simulink library "qss_tb_library"  (Simulink 10.0)
settings: Solver=ode45  StartTime=0.0  StopTime=1220  RelTol=1e-3
undefined symbols (not defined in the file): automatic_gearbox, cc_done, delta_h_C_air, DiscIntNeverNeededParam, dw_GG_c, eta_EG_map, eta_EM_map, eta_ice, g, h, H_o_m, H_u, i_FC_in, i_FC_max, k1, k2, k3, k4, k_cs, M_air, manual_gearbox, P_aux, P_CE_cutoff, P_CE_idle, P_CE_recup, P_CVT_opt, Q_BT_min, Q_SC_IC, r, rho, rho_f, t_c, T_CE_cutoff, T_CE_max, T_EG_c, T_EG_max, T_EM_max, theta_CE, theta_EM, V_CE_map, V_FC_out, w_CE_idle, w_CE_max, w_CE_upper, w_CVT_opt, w_EG_row, w_EG_upper, w_EM_row, w_EM_upper, w_GG_c
(part 2 of 4)

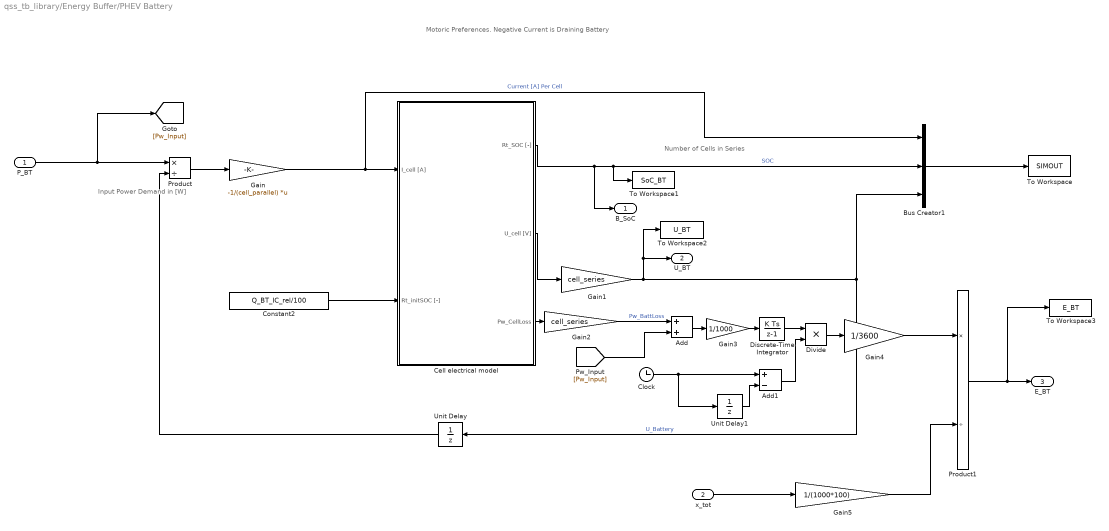
== system qss_tb_library/Energy Buffer/PHEV Battery ==
  note: Number of Cells in Series
  note: Motoric Preferences. Negative Current is Draining Battery
  note: Input Power Demand in [W]
  P_BT : Inport
  x_tot : Inport  Port=2
  Add : Sum
  Add1 : Sum  Inputs=+-
  Bus Creator1 : BusCreator  Inputs=3
  Cell electrical model : Subsystem
  Clock : Clock
  Constant2 : Constant  Value=Q_BT_IC_rel/100
  Discrete-Time Integrator : DiscreteIntegrator  ICPrevOutput=DiscIntNeverNeededParam  ICPrevScaledInput=DiscIntNeverNeededParam
  Divide : Product  Inputs=**
  Gain : Gain  Gain=-1/(cell_parallel)  Multiplication=Matrix(K*u)
  Gain1 : Gain  Gain=cell_series
  Gain2 : Gain  Gain=cell_series
  Gain3 : Gain  Gain=1/1000
  Gain4 : Gain  Gain=1/3600
  Gain5 : Gain  Gain=1/(1000*100)
  Product : Product  Inputs=*/  RndMeth=Zero
  Product1 : Product  Inputs=*/  SaturateOnIntegerOverflow=on  RndMeth=Zero  InputSameDT=on  OutDataTypeStr=Inherit: Same as first input
  To Workspace : ToWorkspace  VariableName=SIMOUT  SaveFormat=Structure With Time  SampleTime=-1
  To Workspace1 : ToWorkspace  VariableName=SoC_BT  SampleTime=-1
      settings: RequirementInfo={} %GIDa_c6642060_f8db_4366_a618_aa68098668f7
  To Workspace2 : ToWorkspace  VariableName=U_BT  SampleTime=-1
      settings: RequirementInfo={} %GIDa_32590376_96d5_473d_a7bc_23059799ede8
  To Workspace3 : ToWorkspace  VariableName=E_BT  SampleTime=-1
  Unit Delay : UnitDelay  InitialCondition=4.07*cell_series  HasFrameUpgradeWarning=on
  Unit Delay1 : UnitDelay  HasFrameUpgradeWarning=on
  B_SoC : Outport  InitialOutput=0
  U_BT : Outport  Port=2  InitialOutput=0
  E_BT : Outport  Port=3  InitialOutput=0
  wires:
  Add1/1 -> Divide/2
  Unit Delay1/1 -> Add1/2
  Clock/1 -> Add1/1, Unit Delay1/1
  Bus Creator1/1 -> To Workspace/1
  Discrete-Time Integrator/1 -> Divide/1
  x_tot/1 -> Gain5/1
  Gain5/1 -> Product1/2
  Gain4/1 -> Product1/1
  Divide/1 -> Gain4/1
  Gain3/1 -> Discrete-Time Integrator/1
  Add/1 -> Gain3/1
  [Pw_Input] -> Add/2
  Gain2/1 -> Add/1  "Pw_BattLoss"
  Cell electrical model/3(Pw_CellLoss) -> Gain2/1
  Product1/1 -> E_BT/1, To Workspace3/1
  P_BT/1 -> Product/1, [Pw_Input]
  Cell electrical model/1(Rt_SOC [-]) -> Bus Creator1/2, To Workspace1/1, B_SoC/1  "SOC"
  Unit Delay/1 -> Product/2
  Product/1 -> Gain/1
  Constant2/1 -> Cell electrical model/2(Rt_initSOC [-])
  Gain1/1 -> Unit Delay/1, Bus Creator1/3, U_BT/1, To Workspace2/1  "U_Battery"
  Cell electrical model/2(U_cell [V]) -> Gain1/1
  Gain/1 -> Cell electrical model/1(I_cell [A]), Bus Creator1/1  "Current [A] Per Cell"

== system qss_tb_library/Energy Buffer/Supercapacitor ==
  P_SC : Inport
  Fcn : Fcn  Expr=(-u[2]/C_SC+sqrt(u[2]^2/C_SC^2-4*R_SC*u[1]))/(2*R_SC)
  Gain : Gain  Gain=1/C_SC  SaturateOnIntegerOverflow=on  OutDataTypeStr=Inherit: Same as input  ParamDataTypeStr=Inherit: Same as input
  Gain1 : Gain  Gain=h  SaturateOnIntegerOverflow=on  OutDataTypeStr=Inherit: Same as input  ParamDataTypeStr=Inherit: Same as input
  Mux : Mux  Inputs=2
  SC charge : UnitDelay  InitialCondition=Q_SC_IC  SampleTime=h  HasFrameUpgradeWarning=on
  Sum3 : Sum  SaturateOnIntegerOverflow=on  InputSameDT=on  OutDataTypeStr=Inherit: Same as first input
  Supervision supercap : Subsystem
  To Workspace1 : ToWorkspace  VariableName=I_SC  SampleTime=1
  To Workspace2 : ToWorkspace  VariableName=U_SC  SampleTime=1
  To Workspace3 : ToWorkspace  VariableName=Q_SC  SampleTime=1
  To Workspace4 : ToWorkspace  VariableName=P_SC  SampleTime=1
  U_SC : Outport  InitialOutput=0
  wires:
  P_SC/1 -> Supervision supercap/2(P_SC), Mux/1, To Workspace4/1
  Gain/1 -> To Workspace2/1, U_SC/1
  Fcn/1 -> To Workspace1/1, Gain1/1
  SC charge/1 -> To Workspace3/1, Supervision supercap/1(Q_SC), Mux/2, Gain/1, Sum3/2
  Sum3/1 -> SC charge/1
  Mux/1 -> Fcn/1
  Gain1/1 -> Sum3/1

== system qss_tb_library/Energy Converter/CE Assignment ==
  w_gear : Inport
  dw_dt_gear : Inport  Port=2
  T_gear : Inport  Port=3
  Constant1 : Constant  Value=P_aux
  Detect fuel cutoff : Subsystem
  Detect idle : Subsystem
  Detect overload and overspeed : Subsystem
  "Engine consumption map V = f(w, T) [kg/s]" : Lookup2D  RowIndex=w_CE_row  ColumnIndex=T_CE_col  Table=V_CE_map
  Engine inertia : Gain  Gain=theta_CE  SaturateOnIntegerOverflow=on  OutDataTypeStr=Inherit: Same as input  ParamDataTypeStr=Inherit: Same as input
  Fuel lower heating value : Gain  Gain=H_u  SaturateOnIntegerOverflow=on  OutDataTypeStr=Inherit: Same as input  ParamDataTypeStr=Inherit: Same as input
  Lower limit (fuel cutoff) : Saturate  UpperLimit=inf  LowerLimit=T_CE_cutoff
  Lower limit (speed at idle) : Saturate  UpperLimit=inf  LowerLimit=w_CE_idle
  To Workspace3 : ToWorkspace  VariableName=T_CE  SampleTime=-1
  To Workspace4 : ToWorkspace  VariableName=w_CE  SampleTime=-1
  To Workspace5 : ToWorkspace  VariableName=P_CE  SampleTime=-1
  Total power : Sum  SaturateOnIntegerOverflow=on  InputSameDT=on  OutDataTypeStr=Inherit: Same as first input
  Total torque : Sum  SaturateOnIntegerOverflow=on  InputSameDT=on  OutDataTypeStr=Inherit: Same as first input
  P_CE : Outport  InitialOutput=0
  wires:
  Lower limit (fuel cutoff)/1 -> To Workspace3/1, Detect fuel cutoff/2(T_CE), Detect idle/3(T_CE), "Engine consumption map V = f(w, T) [kg/s]"/2, Detect overload and overspeed/2(T_CE)
  Constant1/1 -> Total power/2
  Total power/1 -> To Workspace5/1, P_CE/1
  Detect fuel cutoff/1(P_CE) -> Total power/1
  "Engine consumption map V = f(w, T) [kg/s]"/1 -> Fuel lower heating value/1
  Detect idle/1(P_CE) -> Detect fuel cutoff/1(P_CE_fuel)
  Fuel lower heating value/1 -> Detect idle/1(P_CE_fuel)
  w_gear/1 -> Lower limit (speed at idle)/1
  Lower limit (speed at idle)/1 -> To Workspace4/1, "Engine consumption map V = f(w, T) [kg/s]"/1, Detect idle/2(w_CE), Detect overload and overspeed/1(w_CE)
  Engine inertia/1 -> Total torque/2
  Total torque/1 -> Lower limit (fuel cutoff)/1
  dw_dt_gear/1 -> Engine inertia/1
  T_gear/1 -> Total torque/1

== system qss_tb_library/Energy Converter/Combustion Engine (Willans-approximation  with overload detection) ==
  w_gear : Inport
  dw_dt_gear : Inport  Port=2
  T_gear : Inport  Port=3
  Constant1 : Constant  Value=P_aux
  Detect fuel cutoff : Subsystem
  Detect idle : Subsystem
  Detect overload and overspeed : Subsystem
  Engine efficiency : Subsystem
  Engine inertia : Gain  Gain=theta_CE  SaturateOnIntegerOverflow=on  OutDataTypeStr=Inherit: Same as input  ParamDataTypeStr=Inherit: Same as input
  Lower limit (fuel cutoff) : Saturate  UpperLimit=inf  LowerLimit=T_CE_cutoff
  Lower limit (speed at idle) : Saturate  UpperLimit=inf  LowerLimit=w_CE_idle
  Product : Product  Inputs=**/  SaturateOnIntegerOverflow=on  RndMeth=Zero  InputSameDT=on  OutDataTypeStr=Inherit: Same as first input
  To Workspace1 : ToWorkspace  VariableName=eta_CE  SampleTime=-1
  To Workspace3 : ToWorkspace  VariableName=T_CE  SampleTime=-1
  To Workspace4 : ToWorkspace  VariableName=w_CE  SampleTime=-1
  To Workspace5 : ToWorkspace  VariableName=P_CE  SampleTime=-1
  Total power : Sum  SaturateOnIntegerOverflow=on  InputSameDT=on  OutDataTypeStr=Inherit: Same as first input
  Total torque : Sum  SaturateOnIntegerOverflow=on  InputSameDT=on  OutDataTypeStr=Inherit: Same as first input
  P_CE : Outport  InitialOutput=0
  wires:
  Constant1/1 -> Total power/2
  Total power/1 -> To Workspace5/1, P_CE/1
  Detect fuel cutoff/1(P_CE) -> Total power/1
  Detect idle/1(P_CE) -> Detect fuel cutoff/1(P_CE_fuel)
  Product/1 -> Detect idle/1(P_CE_fuel)
  w_gear/1 -> Lower limit (speed at idle)/1
  Lower limit (speed at idle)/1 -> Detect idle/2(w_CE), Engine efficiency/1(w_CE), Product/1, Detect overload and overspeed/1(w_CE), To Workspace4/1
  Lower limit (fuel cutoff)/1 -> To Workspace3/1, Engine efficiency/2(T_CE), Detect fuel cutoff/2(T_CE), Detect idle/3(T_CE), Product/2, Detect overload and overspeed/2(T_CE)
  Engine inertia/1 -> Total torque/2
  Total torque/1 -> Lower limit (fuel cutoff)/1
  dw_dt_gear/1 -> Engine inertia/1
  T_gear/1 -> Total torque/1
  Engine efficiency/1(eta_CE) -> To Workspace1/1, Product/3

== system qss_tb_library/Energy Converter/Combustion Engine (Willans-approximation) ==
  w_gear : Inport
  dw_dt_gear : Inport  Port=2
  T_gear : Inport  Port=3
  Constant1 : Constant  Value=P_aux
  Detect fuel cutoff : Subsystem
  Detect idle : Subsystem
  Engine efficiency : Subsystem
  Engine inertia : Gain  Gain=theta_CE  SaturateOnIntegerOverflow=on  OutDataTypeStr=Inherit: Same as input  ParamDataTypeStr=Inherit: Same as input
  Lower limit (fuel cutoff) : Saturate  UpperLimit=inf  LowerLimit=T_CE_cutoff
  Lower limit (speed at idle) : Saturate  UpperLimit=inf  LowerLimit=w_CE_idle
  Product : Product  Inputs=**/  SaturateOnIntegerOverflow=on  RndMeth=Zero  InputSameDT=on  OutDataTypeStr=Inherit: Same as first input
  To Workspace1 : ToWorkspace  VariableName=eta_CE  SampleTime=-1
  To Workspace3 : ToWorkspace  VariableName=T_CE  SampleTime=-1
  To Workspace4 : ToWorkspace  VariableName=w_CE  SampleTime=-1
  To Workspace5 : ToWorkspace  VariableName=P_CE  SampleTime=-1
  Total power : Sum  SaturateOnIntegerOverflow=on  InputSameDT=on  OutDataTypeStr=Inherit: Same as first input
  Total torque : Sum  SaturateOnIntegerOverflow=on  InputSameDT=on  OutDataTypeStr=Inherit: Same as first input
  P_CE : Outport  InitialOutput=0
  wires:
  Engine efficiency/1(eta_CE) -> Product/3, To Workspace1/1
  T_gear/1 -> Total torque/1
  dw_dt_gear/1 -> Engine inertia/1
  Total torque/1 -> Lower limit (fuel cutoff)/1
  Engine inertia/1 -> Total torque/2
  Lower limit (fuel cutoff)/1 -> Detect idle/3(T_CE), Detect fuel cutoff/2(T_CE), Engine efficiency/2(T_CE), Product/2, To Workspace3/1
  Lower limit (speed at idle)/1 -> To Workspace4/1, Engine efficiency/1(w_CE), Detect idle/2(w_CE), Product/1
  w_gear/1 -> Lower limit (speed at idle)/1
  Product/1 -> Detect idle/1(P_CE_fuel)
  Detect idle/1(P_CE) -> Detect fuel cutoff/1(P_CE_fuel)
  Detect fuel cutoff/1(P_CE) -> Total power/1
  Total power/1 -> P_CE/1, To Workspace5/1
  Constant1/1 -> Total power/2

== system qss_tb_library/Energy Converter/Combustion Engine (consumption map) ==
  w_gear : Inport
  dw_dt_gear : Inport  Port=2
  T_gear : Inport  Port=3
  Constant1 : Constant  Value=P_aux
  Detect fuel cutoff : Subsystem
  Detect idle : Subsystem
  Detect overload and overspeed : Subsystem
  "Engine consumption map V = f(w, T) [kg/s]" : Lookup2D  RowIndex=w_CE_row  ColumnIndex=T_CE_col  Table=V_CE_map
  Engine inertia : Gain  Gain=theta_CE  SaturateOnIntegerOverflow=on  OutDataTypeStr=Inherit: Same as input  ParamDataTypeStr=Inherit: Same as input
  Fuel lower heating value : Gain  Gain=H_u  SaturateOnIntegerOverflow=on  OutDataTypeStr=Inherit: Same as input  ParamDataTypeStr=Inherit: Same as input
  Lower limit (fuel cutoff) : Saturate  UpperLimit=inf  LowerLimit=T_CE_cutoff
  Lower limit (speed at idle) : Saturate  UpperLimit=inf  LowerLimit=w_CE_idle
  To Workspace3 : ToWorkspace  VariableName=T_CE  SampleTime=-1
  To Workspace4 : ToWorkspace  VariableName=w_CE  SampleTime=-1
  To Workspace5 : ToWorkspace  VariableName=P_CE  SampleTime=-1
  Total power : Sum  SaturateOnIntegerOverflow=on  InputSameDT=on  OutDataTypeStr=Inherit: Same as first input
  Total torque : Sum  SaturateOnIntegerOverflow=on  InputSameDT=on  OutDataTypeStr=Inherit: Same as first input
  P_CE : Outport  InitialOutput=0
  wires:
  T_gear/1 -> Total torque/1
  dw_dt_gear/1 -> Engine inertia/1
  Total torque/1 -> Lower limit (fuel cutoff)/1
  Engine inertia/1 -> Total torque/2
  Lower limit (speed at idle)/1 -> Detect overload and overspeed/1(w_CE), Detect idle/2(w_CE), "Engine consumption map V = f(w, T) [kg/s]"/1, To Workspace4/1
  w_gear/1 -> Lower limit (speed at idle)/1
  Fuel lower heating value/1 -> Detect idle/1(P_CE_fuel)
  Detect idle/1(P_CE) -> Detect fuel cutoff/1(P_CE_fuel)
  "Engine consumption map V = f(w, T) [kg/s]"/1 -> Fuel lower heating value/1
  Detect fuel cutoff/1(P_CE) -> Total power/1
  Total power/1 -> P_CE/1, To Workspace5/1
  Constant1/1 -> Total power/2
  Lower limit (fuel cutoff)/1 -> Detect overload and overspeed/2(T_CE), "Engine consumption map V = f(w, T) [kg/s]"/2, Detect idle/3(T_CE), Detect fuel cutoff/2(T_CE), To Workspace3/1

== system qss_tb_library/Energy Converter/Combustion Engine (ideal) ==
  w_gear : Inport
  dw_dt_gear : Inport  Port=2
  T_gear : Inport  Port=3
  Constant1 : Constant  Value=P_aux
  Efficiency : Gain  Gain=1/eta_ice  SaturateOnIntegerOverflow=on  OutDataTypeStr=Inherit: Same as input  ParamDataTypeStr=Inherit: Same as input
  Engine inertia : Gain  Gain=theta_CE  SaturateOnIntegerOverflow=on  OutDataTypeStr=Inherit: Same as input  ParamDataTypeStr=Inherit: Same as input
  Product : Product  RndMeth=Zero
  To Workspace3 : ToWorkspace  VariableName=T_CE  SampleTime=-1
  To Workspace4 : ToWorkspace  VariableName=w_CE  SampleTime=-1
  To Workspace5 : ToWorkspace  VariableName=P_CE  SampleTime=-1
  Total power : Sum  Inputs=+++  SaturateOnIntegerOverflow=on  InputSameDT=on  OutDataTypeStr=Inherit: Same as first input
  Total torque : Sum  SaturateOnIntegerOverflow=on  InputSameDT=on  OutDataTypeStr=Inherit: Same as first input
  "idle -> inf" : Saturate  UpperLimit=inf  LowerLimit=P_CE_idle
  recuperation : Saturate  UpperLimit=0  LowerLimit=P_CE_recup
  P_CE : Outport  InitialOutput=0
  wires:
  recuperation/1 -> Total power/3
  "idle -> inf"/1 -> Efficiency/1
  Constant1/1 -> Total power/2
  Total power/1 -> To Workspace5/1, P_CE/1
  Efficiency/1 -> Total power/1
  Product/1 -> recuperation/1, "idle -> inf"/1
  w_gear/1 -> To Workspace4/1, Product/1
  Engine inertia/1 -> Total torque/2
  Total torque/1 -> To Workspace3/1, Product/2
  dw_dt_gear/1 -> Engine inertia/1
  T_gear/1 -> Total torque/1

== system qss_tb_library/Energy Converter/EG Assignment ==
  w_gear : Inport
  T_gear : Inport  Port=2
  Detect overload and overspeed : Subsystem
  "Efficiency eta = f(w, T)" : Lookup2D  RowIndex=w_EG_row  ColumnIndex=T_EG_col  Table=eta_EG_map
  Product : Product  Inputs=3  SaturateOnIntegerOverflow=on  RndMeth=Zero  InputSameDT=on  OutDataTypeStr=Inherit: Same as first input
  To Workspace1 : ToWorkspace  VariableName=w_EG  SampleTime=-1
  To Workspace2 : ToWorkspace  VariableName=T_EG  SampleTime=-1
  To Workspace5 : ToWorkspace  VariableName=P_EG  SampleTime=-1
  P_EG : Outport  InitialOutput=0
  wires:
  T_gear/1 -> Product/2, "Efficiency eta = f(w, T)"/2, Detect overload and overspeed/2(T_EG), To Workspace2/1
  "Efficiency eta = f(w, T)"/1 -> Product/1
  Product/1 -> P_EG/1, To Workspace5/1
  w_gear/1 -> Product/3, "Efficiency eta = f(w, T)"/1, Detect overload and overspeed/1(w_EG), To Workspace1/1

== system qss_tb_library/Energy Converter/EM Assignment ==
  w_gear : Inport
  dw_dt_gear : Inport  Port=2
  T_gear : Inport  Port=3
  Constant1 : Constant  Value=P_aux
  Detect overload and overspeed : Subsystem
  "Efficiency eta = f(w, T)" : Lookup2D  RowIndex=w_EM_row  ColumnIndex=T_EM_col  Table=eta_EM_map
  Gain1 : Gain  Gain=theta_EM  SaturateOnIntegerOverflow=on  OutDataTypeStr=Inherit: Same as input  ParamDataTypeStr=Inherit: Same as input
  Product : Product  Inputs=3  SaturateOnIntegerOverflow=on  RndMeth=Zero  InputSameDT=on  OutDataTypeStr=Inherit: Same as first input
  To Workspace1 : ToWorkspace  VariableName=w_EM  SampleTime=-1
  To Workspace2 : ToWorkspace  VariableName=T_EM  SampleTime=-1
  To Workspace5 : ToWorkspace  VariableName=P_EM  SampleTime=-1
  Total power : Sum  SaturateOnIntegerOverflow=on  InputSameDT=on  OutDataTypeStr=Inherit: Same as first input
  Total torque : Sum  SaturateOnIntegerOverflow=on  InputSameDT=on  OutDataTypeStr=Inherit: Same as first input
  P_EM : Outport  InitialOutput=0
  wires:
  w_gear/1 -> Detect overload and overspeed/1(w_EM), "Efficiency eta = f(w, T)"/1, Product/3, To Workspace1/1
  "Efficiency eta = f(w, T)"/1 -> Product/1
  dw_dt_gear/1 -> Gain1/1
  T_gear/1 -> Total torque/2
  Gain1/1 -> Total torque/1
  Total torque/1 -> Detect overload and overspeed/2(T_EM), "Efficiency eta = f(w, T)"/2, Product/2, To Workspace2/1
  Constant1/1 -> Total power/2
  Product/1 -> Total power/1
  Total power/1 -> P_EM/1, To Workspace5/1

== system qss_tb_library/Energy Converter/Electric Generator ==
  w_gear : Inport
  T_gear : Inport  Port=2
  Detect overload and overspeed : Subsystem
  "Efficiency eta = f(w, T)" : Lookup2D  RowIndex=w_EG_row  ColumnIndex=T_EG_col  Table=eta_EG_map
  Product : Product  Inputs=3  SaturateOnIntegerOverflow=on  RndMeth=Zero  InputSameDT=on  OutDataTypeStr=Inherit: Same as first input
  To Workspace1 : ToWorkspace  VariableName=w_EG  SampleTime=-1
  To Workspace2 : ToWorkspace  VariableName=T_EG  SampleTime=-1
  To Workspace5 : ToWorkspace  VariableName=P_EG  SampleTime=-1
  P_EG : Outport  InitialOutput=0
  wires:
  T_gear/1 -> Product/2, "Efficiency eta = f(w, T)"/2, Detect overload and overspeed/2(T_EG), To Workspace2/1
  "Efficiency eta = f(w, T)"/1 -> Product/1
  Product/1 -> P_EG/1, To Workspace5/1
  w_gear/1 -> Product/3, "Efficiency eta = f(w, T)"/1, Detect overload and overspeed/1(w_EG), To Workspace1/1

== system qss_tb_library/Energy Converter/Electric Motor ==
  w_gear : Inport
  dw_dt_gear : Inport  Port=2
  T_gear : Inport  Port=3
  Constant1 : Constant  Value=P_aux
  Detect overload and overspeed : Subsystem
  "Efficiency eta = f(w, T)" : Lookup2D  RowIndex=w_EM_row  ColumnIndex=T_EM_col  Table=eta_EM_map
  Gain1 : Gain  Gain=theta_EM  SaturateOnIntegerOverflow=on  OutDataTypeStr=Inherit: Same as input  ParamDataTypeStr=Inherit: Same as input
  Product : Product  Inputs=3  SaturateOnIntegerOverflow=on  RndMeth=Zero  InputSameDT=on  OutDataTypeStr=Inherit: Same as first input
  To Workspace1 : ToWorkspace  VariableName=w_EM  SampleTime=-1
  To Workspace2 : ToWorkspace  VariableName=T_EM  SampleTime=-1
  To Workspace5 : ToWorkspace  VariableName=P_EM  SampleTime=-1
  Total power : Sum  SaturateOnIntegerOverflow=on  InputSameDT=on  OutDataTypeStr=Inherit: Same as first input
  Total torque : Sum  SaturateOnIntegerOverflow=on  InputSameDT=on  OutDataTypeStr=Inherit: Same as first input
  P_EM : Outport  InitialOutput=0
  wires:
  w_gear/1 -> Detect overload and overspeed/1(w_EM), "Efficiency eta = f(w, T)"/1, Product/3, To Workspace1/1
  "Efficiency eta = f(w, T)"/1 -> Product/1
  dw_dt_gear/1 -> Gain1/1
  T_gear/1 -> Total torque/2
  Gain1/1 -> Total torque/1
  Total torque/1 -> Detect overload and overspeed/2(T_EM), "Efficiency eta = f(w, T)"/2, Product/2, To Workspace2/1
  Constant1/1 -> Total power/2
  Product/1 -> Total power/1
  Total power/1 -> P_EM/1, To Workspace5/1

== system qss_tb_library/Energy Converter/Fuel Cell ==
  note: E-Motor is disengaged, as soon as required power
      |  is <= P_fc_idle (->idle speed energy consumption)
  P_in : Inport
  Compressor with E-motor : Subsystem
  Constant3 : Constant  Value=P_FC_idle
  Constant4 : Constant  Value=V_th
  Fuel cell model : Lookup  InputValues=i_FC_in  Table=V_FC_out  SaturateOnIntegerOverflow=on
  Heat losses : ToWorkspace  VariableName=P_loss  SampleTime=1
  Product2 : Product  SaturateOnIntegerOverflow=on  RndMeth=Zero  InputSameDT=on  OutDataTypeStr=Inherit: Same as first input
  Product3 : Product  Inputs=/*  SaturateOnIntegerOverflow=on  RndMeth=Zero  InputSameDT=on  OutDataTypeStr=Inherit: Same as first input
  Stack current : Product  Inputs=*/  SaturateOnIntegerOverflow=on  RndMeth=Zero  InputSameDT=on  OutDataTypeStr=Inherit: Same as first input
  Stack voltage : UnitDelay  InitialCondition=10  SampleTime=h  HasFrameUpgradeWarning=on
  Sum : Sum  SaturateOnIntegerOverflow=on  InputSameDT=on  OutDataTypeStr=Inherit: Same as first input
  Sum1 : Sum  Inputs=+-  SaturateOnIntegerOverflow=on  InputSameDT=on  OutDataTypeStr=Inherit: Same as first input
  Supervision of current density : Subsystem
  Switch1 : Switch  Threshold=P_FC_idle  SaturateOnIntegerOverflow=on  InputSameDT=on
  Theoretical cell voltage : Gain  Gain=1/V_th  SaturateOnIntegerOverflow=on  OutDataTypeStr=Inherit: Same as input  ParamDataTypeStr=Inherit: Same as input
  To Workspace2 : ToWorkspace  VariableName=V_FC  SampleTime=1
  To Workspace4 : ToWorkspace  VariableName=I_FC  SampleTime=1
  To Workspace5 : ToWorkspace  VariableName=i_FC  SampleTime=1
  To Workspace7 : ToWorkspace  VariableName=P_FC  SampleTime=1
  "[A/m^2]" : Gain  Gain=1/A_FC  SaturateOnIntegerOverflow=on  OutDataTypeStr=Inherit: Same as input  ParamDataTypeStr=Inherit: Same as input
  stack number : Gain  Gain=N_FC  SaturateOnIntegerOverflow=on  OutDataTypeStr=Inherit: Same as input  ParamDataTypeStr=Inherit: Same as input
  stack number1 : Gain  Gain=N_FC  SaturateOnIntegerOverflow=on  OutDataTypeStr=Inherit: Same as input  ParamDataTypeStr=Inherit: Same as input
  P_FC : Outport  InitialOutput=0
  wires:
  Compressor with E-motor/1(P_EM_C) -> Sum/2
  Switch1/1 -> Stack current/1, Product3/2
  Constant3/1 -> Switch1/3
  Sum/1 -> Switch1/2, Switch1/1
  P_in/1 -> Sum/1
  Constant4/1 -> Sum1/1
  stack number/1 -> Stack voltage/1
  Sum1/1 -> stack number1/1
  stack number1/1 -> Product2/2
  "[A/m^2]"/1 -> Fuel cell model/1, To Workspace5/1, Supervision of current density/1("   i_FC")
  Theoretical cell voltage/1 -> Product3/1
  Fuel cell model/1 -> stack number/1, Sum1/2, Theoretical cell voltage/1
  Stack current/1 -> "[A/m^2]"/1, Product2/1, To Workspace4/1
  Stack voltage/1 -> Stack current/2, To Workspace2/1
  Product3/1 -> P_FC/1, To Workspace7/1, Compressor with E-motor/1(P_FC)
  Product2/1 -> Heat losses/1

== system qss_tb_library/Energy Source/Tank ==
  P_fuel : Inport
  x_tot : Inport  Port=2
  Factor for cold start : Gain  Gain=k_cs  SaturateOnIntegerOverflow=on  OutDataTypeStr=Inherit: Same as input  ParamDataTypeStr=Inherit: Same as input
  Fu2131el density : Gain  Gain=1/rho_f  SaturateOnIntegerOverflow=on  OutDataTypeStr=Inherit: Same as input  ParamDataTypeStr=Inherit: Same as input
  Gain3 : Gain  Gain=1e5  SaturateOnIntegerOverflow=on  OutDataTypeStr=Inherit: Same as input  ParamDataTypeStr=Inherit: Same as input
  Integration : Subsystem
  Product : Product  Inputs=*/  SaturateOnIntegerOverflow=on  RndMeth=Zero  InputSameDT=on  OutDataTypeStr=Inherit: Same as first input
  To Workspace7 : ToWorkspace  VariableName=V_liter  SampleTime=-1
  liter/100 km : Outport  InitialOutput=0
  wires:
  P_fuel/1 -> Integration/1(P_fuel)
  x_tot/1 -> Product/2
  Integration/1(m_fuel) -> Fu2131el density/1
  Gain3/1 -> liter/100 km/1, To Workspace7/1
  Fu2131el density/1 -> Product/1
  Product/1 -> Factor for cold start/1
  Factor for cold start/1 -> Gain3/1

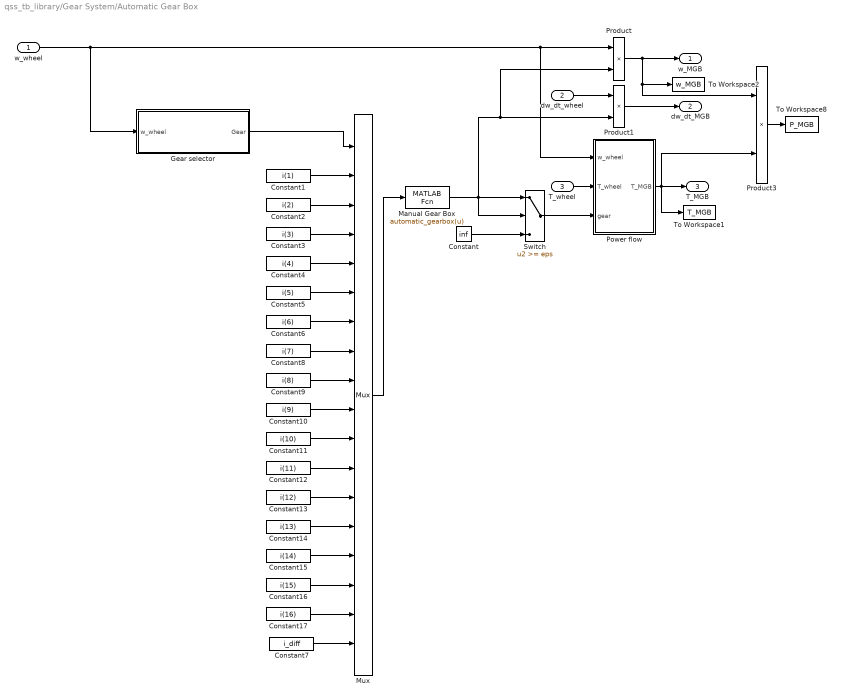
== system qss_tb_library/Gear System/Automatic Gear Box ==
  w_wheel : Inport
  dw_dt_wheel : Inport  Port=2
  T_wheel : Inport  Port=3
  Constant : Constant  Value=inf
  Constant1 : Constant  Value=i(1)
  Constant10 : Constant  Value=i(9)
  Constant11 : Constant  Value=i(10)
  Constant12 : Constant  Value=i(11)
  Constant13 : Constant  Value=i(12)
  Constant14 : Constant  Value=i(13)
  Constant15 : Constant  Value=i(14)
  Constant16 : Constant  Value=i(15)
  Constant17 : Constant  Value=i(16)
  Constant2 : Constant  Value=i(2)
  Constant3 : Constant  Value=i(3)
  Constant4 : Constant  Value=i(4)
  Constant5 : Constant  Value=i(5)
  Constant6 : Constant  Value=i(6)
  Constant7 : Constant  Value=i_diff
  Constant8 : Constant  Value=i(7)
  Constant9 : Constant  Value=i(8)
  Gear selector : Subsystem
  Manual Gear Box : MATLABFcn  MATLABFcn=automatic_gearbox(u)  OutputDimensions=1
  Mux : Mux  Inputs=18
  Power flow : Subsystem
  Product : Product  SaturateOnIntegerOverflow=on  RndMeth=Zero  InputSameDT=on  OutDataTypeStr=Inherit: Same as first input
  Product1 : Product  SaturateOnIntegerOverflow=on  RndMeth=Zero  InputSameDT=on  OutDataTypeStr=Inherit: Same as first input
  Product3 : Product  SaturateOnIntegerOverflow=on  RndMeth=Zero  InputSameDT=on  OutDataTypeStr=Inherit: Same as first input
  Switch : Switch  Threshold=eps  SaturateOnIntegerOverflow=on  InputSameDT=on
  To Workspace1 : ToWorkspace  VariableName=T_MGB  SampleTime=-1
  To Workspace2 : ToWorkspace  VariableName=w_MGB  SampleTime=-1
  To Workspace8 : ToWorkspace  VariableName=P_MGB  SampleTime=-1
  w_MGB : Outport  InitialOutput=0
  dw_dt_MGB : Outport  Port=2  InitialOutput=0
  T_MGB : Outport  Port=3  InitialOutput=0
  wires:
  Mux/1 -> Manual Gear Box/1
  Gear selector/1(Gear) -> Mux/1
  Constant6/1 -> Mux/7
  Constant5/1 -> Mux/6
  Constant4/1 -> Mux/5
  Constant3/1 -> Mux/4
  Constant2/1 -> Mux/3
  Constant1/1 -> Mux/2
  T_wheel/1 -> Power flow/2(T_wheel)
  Switch/1 -> Power flow/3(gear)
  Product3/1 -> To Workspace8/1
  Manual Gear Box/1 -> Switch/1, Switch/2, Product1/2, Product/2
  dw_dt_wheel/1 -> Product1/1
  Product1/1 -> dw_dt_MGB/1
  w_wheel/1 -> Power flow/1(w_wheel), Product/1, Gear selector/1(w_wheel)
  Constant/1 -> Switch/3
  Product/1 -> To Workspace2/1, Product3/1, w_MGB/1
  Power flow/1(T_MGB) -> To Workspace1/1, Product3/2, T_MGB/1
  Constant7/1 -> Mux/18
  Constant8/1 -> Mux/8
  Constant9/1 -> Mux/9
  Constant10/1 -> Mux/10
  Constant11/1 -> Mux/11
  Constant12/1 -> Mux/12
  Constant13/1 -> Mux/13
  Constant14/1 -> Mux/14
  Constant15/1 -> Mux/15
  Constant16/1 -> Mux/16
  Constant17/1 -> Mux/17

== system qss_tb_library/Gear System/Continuously Variable Transmission ==
  w_wheel : Inport
  dw_dt_wheel : Inport  Port=2
  T_wheel : Inport  Port=3
  j_CVT : Inport  Port=4
  dj_CVT : Inport  Port=5
  Power flow : Subsystem
  Product{,1..3} (4 alike) : Product  SaturateOnIntegerOverflow=on  RndMeth=Zero  InputSameDT=on  OutDataTypeStr=Inherit: Same as first input
  Sum : Sum  SaturateOnIntegerOverflow=on  InputSameDT=on  OutDataTypeStr=Inherit: Same as first input
  To Workspace1 : ToWorkspace  VariableName=w_CVT  SampleTime=-1
  To Workspace8 : ToWorkspace  VariableName=P_CVT  SampleTime=-1
  To Workspace9 : ToWorkspace  VariableName=T_CVT  SampleTime=-1
  w_CVT : Outport  InitialOutput=0
  dw_dt_CVT : Outport  Port=2  InitialOutput=0
  T_CVT : Outport  Port=3  InitialOutput=0
  wires:
  w_wheel/1 -> Power flow/1(w_wheel), Product2/1, Product/1
  Power flow/1(T_CVT) -> To Workspace9/1, T_CVT/1, Product3/2
  Product/1 -> Product3/1, w_CVT/1, To Workspace1/1
  Sum/1 -> dw_dt_CVT/1
  dw_dt_wheel/1 -> Product1/1
  dj_CVT/1 -> Product2/2
  j_CVT/1 -> Product1/2, Product/2, Power flow/3(j_CVT)
  Product1/1 -> Sum/2
  Product2/1 -> Sum/1
  T_wheel/1 -> Power flow/2(T_wheel)
  Product3/1 -> To Workspace8/1

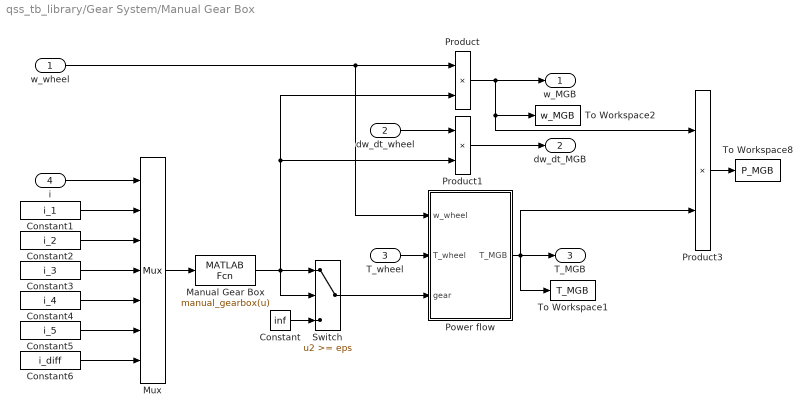
== system qss_tb_library/Gear System/Manual Gear Box ==
  w_wheel : Inport
  dw_dt_wheel : Inport  Port=2
  T_wheel : Inport  Port=3
  i : Inport  Port=4
  Constant : Constant  Value=inf
  Constant1 : Constant  Value=i_1
  Constant2 : Constant  Value=i_2
  Constant3 : Constant  Value=i_3
  Constant4 : Constant  Value=i_4
  Constant5 : Constant  Value=i_5
  Constant6 : Constant  Value=i_diff
  Manual Gear Box : MATLABFcn  MATLABFcn=manual_gearbox(u)  OutputDimensions=1
  Mux : Mux  Inputs=7
  Power flow : Subsystem
  Product : Product  SaturateOnIntegerOverflow=on  RndMeth=Zero  InputSameDT=on  OutDataTypeStr=Inherit: Same as first input
  Product1 : Product  SaturateOnIntegerOverflow=on  RndMeth=Zero  InputSameDT=on  OutDataTypeStr=Inherit: Same as first input
  Product3 : Product  SaturateOnIntegerOverflow=on  RndMeth=Zero  InputSameDT=on  OutDataTypeStr=Inherit: Same as first input
  Switch : Switch  Threshold=eps  SaturateOnIntegerOverflow=on  InputSameDT=on
  To Workspace1 : ToWorkspace  VariableName=T_MGB  SampleTime=-1
  To Workspace2 : ToWorkspace  VariableName=w_MGB  SampleTime=-1
  To Workspace8 : ToWorkspace  VariableName=P_MGB  SampleTime=-1
  w_MGB : Outport  InitialOutput=0
  dw_dt_MGB : Outport  Port=2  InitialOutput=0
  T_MGB : Outport  Port=3  InitialOutput=0
  wires:
  Power flow/1(T_MGB) -> T_MGB/1, Product3/2, To Workspace1/1
  Product/1 -> w_MGB/1, Product3/1, To Workspace2/1
  Constant/1 -> Switch/3
  w_wheel/1 -> Product/1, Power flow/1(w_wheel)
  Product1/1 -> dw_dt_MGB/1
  dw_dt_wheel/1 -> Product1/1
  Manual Gear Box/1 -> Product/2, Product1/2, Switch/2, Switch/1
  Product3/1 -> To Workspace8/1
  Switch/1 -> Power flow/3(gear)
  T_wheel/1 -> Power flow/2(T_wheel)
  Constant1/1 -> Mux/2
  Constant2/1 -> Mux/3
  Constant3/1 -> Mux/4
  Constant4/1 -> Mux/5
  Constant5/1 -> Mux/6
  Constant6/1 -> Mux/7
  i/1 -> Mux/1
  Mux/1 -> Manual Gear Box/1

== system qss_tb_library/Gear System/Simple Transmission ==
  w_wheel : Inport
  dw_dt_wheel : Inport  Port=2
  t_wheel : Inport  Port=3
  Constant : Constant  Value=gear_ratio
  Power flow : Subsystem
  Product : Product  SaturateOnIntegerOverflow=on  RndMeth=Zero  InputSameDT=on  OutDataTypeStr=Inherit: Same as first input
  Product1 : Product  SaturateOnIntegerOverflow=on  RndMeth=Zero  InputSameDT=on  OutDataTypeStr=Inherit: Same as first input
  Product3 : Product  SaturateOnIntegerOverflow=on  RndMeth=Zero  InputSameDT=on  OutDataTypeStr=Inherit: Same as first input
  To Workspace1 : ToWorkspace  VariableName=w_trans  SampleTime=-1
  To Workspace2 : ToWorkspace  VariableName=T_trans  SampleTime=-1
  To Workspace3 : ToWorkspace  VariableName=P_trans  SampleTime=-1
  w_trans : Outport  InitialOutput=0
  dw_dt_trans : Outport  Port=2  InitialOutput=0
  T_trans : Outport  Port=3  InitialOutput=0
  wires:
  Product3/1 -> To Workspace3/1
  Constant/1 -> Product/2, Product1/2, Power flow/3(gear_ratio)
  dw_dt_wheel/1 -> Product1/1
  Product/1 -> Product3/1, To Workspace1/1, w_trans/1
  Product1/1 -> dw_dt_trans/1
  Power flow/1(T_trans) -> Product3/2, To Workspace2/1, T_trans/1
  w_wheel/1 -> Power flow/1(w_wheel), Product/1
  t_wheel/1 -> Power flow/2(T_wheel)

== system qss_tb_library/Gear System/Simple Transmission2 ==
  w_wheel : Inport
  dw_dt_wheel : Inport  Port=2
  T_wheel : Inport  Port=3
  Product3 : Product  SaturateOnIntegerOverflow=on  RndMeth=Zero  InputSameDT=on  OutDataTypeStr=Inherit: Same as first input
  To Workspace1 : ToWorkspace  VariableName=w_trans  SampleTime=-1
  To Workspace2 : ToWorkspace  VariableName=T_trans  SampleTime=-1
  To Workspace3 : ToWorkspace  VariableName=P_trans  SampleTime=-1
  w_trans : Outport  InitialOutput=0
  dw_dt_trans : Outport  Port=2  InitialOutput=0
  T_trans : Outport  Port=3  InitialOutput=0
  wires:
  dw_dt_wheel/1 -> dw_dt_trans/1
  T_wheel/1 -> To Workspace2/1, T_trans/1, Product3/2
  w_wheel/1 -> w_trans/1, Product3/1, To Workspace1/1
  Product3/1 -> To Workspace3/1

== system qss_tb_library/Vehicle/Simple wheel model ==
  v_veh : Inport
  a_veh : Inport  Port=2
  F_Trac : Inport  Port=3
  Gain1 : Gain  Gain=1/(0.5*d_wheel)  SaturateOnIntegerOverflow=on  OutDataTypeStr=Inherit: Same as input  ParamDataTypeStr=Inherit: Same as input
  Gain2 : Gain  Gain=1/(0.5*d_wheel)  SaturateOnIntegerOverflow=on  OutDataTypeStr=Inherit: Same as input  ParamDataTypeStr=Inherit: Same as input
  Gain3 : Gain  Gain=0.5*d_wheel  SaturateOnIntegerOverflow=on  OutDataTypeStr=Inherit: Same as input  ParamDataTypeStr=Inherit: Same as input
  To Workspace1 : ToWorkspace  VariableName=w_wheel  SampleTime=-1
  To Workspace2 : ToWorkspace  VariableName=T_wheel  SampleTime=-1
  To Workspace3 : ToWorkspace  VariableName=dw_dt_wheel  SampleTime=-1
  w_wheel : Outport  InitialOutput=0
  dw_dt_wheel : Outport  Port=2  InitialOutput=0
  T_wheel : Outport  Port=3  InitialOutput=0
  wires:
  Gain2/1 -> dw_dt_wheel/1, To Workspace3/1
  Gain1/1 -> w_wheel/1, To Workspace1/1
  Gain3/1 -> To Workspace2/1, T_wheel/1
  a_veh/1 -> Gain2/1
  F_Trac/1 -> Gain3/1
  v_veh/1 -> Gain1/1

== system qss_tb_library/Vehicle/Vehicle ==
  v : Inport
  a : Inport  Port=2
  alfa : Inport  Port=3
  Acceleration Force : Subsystem
  Aerodynamic resistance : Subsystem
  Average speed : Subsystem
  Gain1 : Gain  Gain=1+k_inertia/100  SaturateOnIntegerOverflow=on  OutDataTypeStr=Inherit: Same as input  ParamDataTypeStr=Inherit: Same as input
  Required Traction force : Sum  Inputs=++++  SaturateOnIntegerOverflow=on  InputSameDT=on  OutDataTypeStr=Inherit: Same as first input
  Rolling resistance : Subsystem
  To Workspace1 : ToWorkspace  VariableName=v_veh  SampleTime=-1
  To Workspace2 : ToWorkspace  VariableName=F_grade  SampleTime=-1
  To Workspace3 : ToWorkspace  VariableName=a_veh  SampleTime=-1
  To Workspace5 : ToWorkspace  VariableName=F_roll  SampleTime=-1
  To Workspace6 : ToWorkspace  VariableName=F_Trac  SampleTime=-1
  To Workspace8 : ToWorkspace  VariableName=F_net  SampleTime=-1
  To Workspace9 : ToWorkspace  VariableName=F_aero  SampleTime=-1
  gradient force : Subsystem
  v_veh : Outport  InitialOutput=0
  a_veh : Outport  Port=2  InitialOutput=0
  F_Trac : Outport  Port=3  InitialOutput=0
  wires:
  Gain1/1 -> Required Traction force/3, To Workspace8/1
  gradient force/1(F_grade) -> To Workspace2/1, Required Traction force/4
  alfa/1 -> gradient force/1(alfa), Rolling resistance/2(alfa)
  Required Traction force/1 -> F_Trac/1, To Workspace6/1
  Acceleration Force/1(F_Net) -> Gain1/1
  Aerodynamic resistance/1(F_aero) -> To Workspace9/1, Required Traction force/2
  Rolling resistance/1(F_roll) -> To Workspace5/1, Required Traction force/1
  a/1 -> Acceleration Force/1(a_veh), To Workspace3/1, a_veh/1
  v/1 -> Average speed/1(v)
  Average speed/1(v_a) -> Aerodynamic resistance/1(v), Rolling resistance/1(v), v_veh/1, To Workspace1/1

== system qss_tb_library/Controller/Battery Controller/Geno-Group On ==
  cc_on : Inport
  Clock : Subsystem  mask(Digital clock){Parameter2=2}
      mask prompts: Parameter2 "Period:"
      mask help:
      | Digital clock.
      | Output is set to 1 for the first half of the period.
      mask init:
      | duration = @1/2;
      mask Help: Digital clock for logic systems.
      mask Display: plot(0,0,100,100,[90,75,75,60,60,35,35,20,20,10],[20,20,80,80,19,20,80,80,20,20])
  Constant : Constant  Value=cc_done
  Counter : UnitDelay  SampleTime=h  HasFrameUpgradeWarning=on
  Data Type Conversion1 : DataTypeConversion  OutDataTypeStr=boolean
  Data Type Conversion2 : DataTypeConversion  OutDataTypeStr=double
  Data Type Conversion3 : DataTypeConversion  OutDataTypeStr=double
  Logical operator3 : Logic
  Mux : Mux  Inputs=3
  Product : Product  SaturateOnIntegerOverflow=on  RndMeth=Zero  InputSameDT=on  OutDataTypeStr=Inherit: Same as first input
  Relational Operator : RelationalOperator  OutDataTypeStr=boolean  RndMeth=Nearest  InputSameDT=on
  Sum3 : Sum  Inputs=++-  SaturateOnIntegerOverflow=on  InputSameDT=on  OutDataTypeStr=Inherit: Same as first input
  T_EG start-up : Lookup  InputValues=t_c  Table=T_EG_c  SaturateOnIntegerOverflow=on
  dw start-up : Lookup  InputValues=t_c  Table=dw_GG_c  SaturateOnIntegerOverflow=on
  w start-up : Lookup  InputValues=t_c  Table=w_GG_c  SaturateOnIntegerOverflow=on
  OutOn : Outport  InitialOutput=0
  done : Outport  Port=2  InitialOutput=0
  wires:
  Data Type Conversion3/1 -> Product/1
  Data Type Conversion2/1 -> Sum3/2
  Data Type Conversion1/1 -> Logical operator3/2
  Mux/1 -> OutOn/1
  T_EG start-up/1 -> Mux/3
  dw start-up/1 -> Mux/2
  w start-up/1 -> Mux/1
  Logical operator3/1 -> Data Type Conversion2/1
  Counter/1 -> Sum3/1, dw start-up/1, T_EG start-up/1, Product/2, Relational Operator/1, w start-up/1
  Sum3/1 -> Counter/1
  Clock/1(out_1) -> Data Type Conversion1/1
  cc_on/1 -> Logical operator3/1
  Product/1 -> Sum3/3
  Constant/1 -> Relational Operator/2
  Relational Operator/1 -> Data Type Conversion3/1, done/1

== system qss_tb_library/Controller/Battery Controller/S-R Flip-Flop ==
  S : Inport
  R : Inport  Port=2
  Demux : Demux  Outputs=2
  Logic : CombinatorialLogic  TruthTable=[0 1;0 1;1 0;0 1;1 0;0 1;1 0;1 0]
  Memory : Memory  InheritSampleTime=on
  Mux : Mux  Inputs=3
  Q : Outport  InitialOutput=0
  !Q : Outport  Port=2  InitialOutput=1
  wires:
  R/1 -> Mux/3
  S/1 -> Mux/2
  Memory/1 -> Mux/1
  Demux/1 -> Memory/1, Q/1
  Demux/2 -> !Q/1
  Logic/1 -> Demux/1
  Mux/1 -> Logic/1

== system qss_tb_library/Driving Cycle/Driving Cycle/Differentiation ==
  V_z : Inport
  Sum1 : Sum  Inputs=+-  SaturateOnIntegerOverflow=on  InputSameDT=on  OutDataTypeStr=Inherit: Same as first input
  Unit Delay1 : UnitDelay  SampleTime=h  HasFrameUpgradeWarning=on
  D_z : Outport  InitialOutput=0
  wires:
  Sum1/1 -> D_z/1
  V_z/1 -> Unit Delay1/1, Sum1/1
  Unit Delay1/1 -> Sum1/2

== system qss_tb_library/Driving Cycle/Driving Cycle/Integration ==
  V_z : Inport
  Gain4 : Gain  Gain=0.5*h  SaturateOnIntegerOverflow=on  OutDataTypeStr=Inherit: Same as input  ParamDataTypeStr=Inherit: Same as input
  Plant : UnitDelay  InitialCondition=1  SampleTime=h  HasFrameUpgradeWarning=on
  Sum2 : Sum  SaturateOnIntegerOverflow=on  InputSameDT=on  OutDataTypeStr=Inherit: Same as first input
  Sum4 : Sum  SaturateOnIntegerOverflow=on  InputSameDT=on  OutDataTypeStr=Inherit: Same as first input
  Unit Delay2 : UnitDelay  SampleTime=h  HasFrameUpgradeWarning=on
  x_tot : Outport  InitialOutput=0
  wires:
  Plant/1 -> x_tot/1, Sum4/1
  Sum4/1 -> Plant/1
  Gain4/1 -> Sum4/2
  V_z/1 -> Unit Delay2/1, Sum2/1
  Unit Delay2/1 -> Sum2/2
  Sum2/1 -> Gain4/1

== system qss_tb_library/Driving Cycle/Driving Cycle  (with performance  test possibility)/Differentiation ==
  V_z : Inport
  Sum1 : Sum  Inputs=+-  SaturateOnIntegerOverflow=on  InputSameDT=on  OutDataTypeStr=Inherit: Same as first input
  Unit Delay1 : UnitDelay  SampleTime=h  HasFrameUpgradeWarning=on
  D_z : Outport  InitialOutput=0
  wires:
  Sum1/1 -> D_z/1
  V_z/1 -> Unit Delay1/1, Sum1/1
  Unit Delay1/1 -> Sum1/2

== system qss_tb_library/Driving Cycle/Driving Cycle  (with performance  test possibility)/Gear selector ==
  speed [m/s] : Inport
  Constant : Constant  Value=0
  Gear1 : Relay  OffSwitchValue=0
  Gear2 : Relay  OnSwitchValue=gearon(1)/3.6  OffSwitchValue=gearoff(1)/3.6
  Gear3 : Relay  OnSwitchValue=gearon(2)/3.6  OffSwitchValue=gearoff(2)/3.6
  Gear4 : Relay  OnSwitchValue=gearon(3)/3.6  OffSwitchValue=gearoff(3)/3.6
  Gear5 : Relay  OnSwitchValue=gearon(4)/3.6  OffSwitchValue=gearoff(4)/3.6
  Sum : Sum  Inputs=5  SaturateOnIntegerOverflow=on
  Sum1 : Sum  Inputs=2  SaturateOnIntegerOverflow=on
  Gear : Outport
  wires:
  Constant/1 -> Sum1/2
  Sum1/1 -> Gear/1
  Sum/1 -> Sum1/1
  Gear4/1 -> Sum/4
  Gear3/1 -> Sum/3
  Gear2/1 -> Sum/2
  Gear1/1 -> Sum/1
  speed [m/s]/1 -> Gear4/1, Gear5/1, Gear3/1, Gear2/1, Gear1/1
  Gear5/1 -> Sum/5

== system qss_tb_library/Driving Cycle/Driving Cycle  (with performance  test possibility)/Integration ==
  V_z : Inport
  Gain4 : Gain  Gain=0.5*h  SaturateOnIntegerOverflow=on  OutDataTypeStr=Inherit: Same as input  ParamDataTypeStr=Inherit: Same as input
  Plant : UnitDelay  InitialCondition=1  SampleTime=h  HasFrameUpgradeWarning=on
  Sum2 : Sum  SaturateOnIntegerOverflow=on  InputSameDT=on  OutDataTypeStr=Inherit: Same as first input
  Sum4 : Sum  SaturateOnIntegerOverflow=on  InputSameDT=on  OutDataTypeStr=Inherit: Same as first input
  Unit Delay2 : UnitDelay  SampleTime=h  HasFrameUpgradeWarning=on
  x_tot : Outport  InitialOutput=0
  wires:
  Plant/1 -> x_tot/1, Sum4/1
  Sum4/1 -> Plant/1
  Gain4/1 -> Sum4/2
  V_z/1 -> Unit Delay2/1, Sum2/1
  Unit Delay2/1 -> Sum2/2
  Sum2/1 -> Gain4/1

== system qss_tb_library/Driving Cycle/Driving Cycle (no gradient)/Differentiation ==
  V_z : Inport
  Sum1 : Sum  Inputs=+-  SaturateOnIntegerOverflow=on  InputSameDT=on  OutDataTypeStr=Inherit: Same as first input
  Unit Delay1 : UnitDelay  SampleTime=h  HasFrameUpgradeWarning=on
  D_z : Outport  InitialOutput=0
  wires:
  Unit Delay1/1 -> Sum1/2
  V_z/1 -> Sum1/1, Unit Delay1/1
  Sum1/1 -> D_z/1

== system qss_tb_library/Driving Cycle/Driving Cycle (no gradient)/Integration ==
  V_z : Inport
  Gain4 : Gain  Gain=0.5*h  SaturateOnIntegerOverflow=on  OutDataTypeStr=Inherit: Same as input  ParamDataTypeStr=Inherit: Same as input
  Plant : UnitDelay  InitialCondition=1  SampleTime=h  HasFrameUpgradeWarning=on
  Sum2 : Sum  SaturateOnIntegerOverflow=on  InputSameDT=on  OutDataTypeStr=Inherit: Same as first input
  Sum4 : Sum  SaturateOnIntegerOverflow=on  InputSameDT=on  OutDataTypeStr=Inherit: Same as first input
  Unit Delay2 : UnitDelay  SampleTime=h  HasFrameUpgradeWarning=on
  x_tot : Outport  InitialOutput=0
  wires:
  Sum2/1 -> Gain4/1
  Unit Delay2/1 -> Sum2/2
  V_z/1 -> Sum2/1, Unit Delay2/1
  Gain4/1 -> Sum4/2
  Sum4/1 -> Plant/1
  Plant/1 -> Sum4/1, x_tot/1

== system qss_tb_library/Energy Buffer/48V Battery/Cell electrical model ==
  I_cell [A] : Inport
  Rt_initSOC [-] : Inport  Port=2
  Add3 : Sum
  DOD->SOC : Fcn  Expr=1-u(1)
  Open-circuit voltage : Lookup  InputValues=[-0.08,-0.03,0,0.005,0.025,0.05,0.085,0.155,0.25,0.3,0.34,0.365,0.395,0.41,0.5,0.52,0.62,0.7,0.73,0.76,0.8,0.82,0.83,0.85,0.89,0.9,0.91,0.92,0.935,0.95,0.965,0.98,0.99,0.995,1,1.011,1.015]  Table=[4.32,4.22,4.15,4.12,4.115,4.1,4.07,4.03,3.96,3.92,3.915,3.8937,3.8622,3.8537,3.7828,3.7672,3.7022,3.6562,3.6398,3.6098,3.4,3.3,3.2,3.18,3.17,3.15,3.1,3.1,3,2.95,2.8437,2.8437,2.8437,2.8437,2.8437,2.5,2]  LookUpMeth=Interpolation-Use End Values
  Product1 : Product  Inputs=**  RndMeth=Zero
  Product2 : Product  Inputs=**  RndMeth=Zero
  Resistance : Lookup  InputValues=[0,0.16666666666666666,0.3333333333333333,0.5,0.6666666666666666,0.8333333333333334,1]  Table=0.25*[0.024012,0.0100,0.0075,0.00375,0.0022500000000000003,0.0015,0.0011250000000000001]
  State of charge calculation : Subsystem
  Stop Function : Subsystem
  Rt_SOC [-] : Outport
  U_cell [V] : Outport  Port=2
  Pw_CellLoss : Outport  Port=3
  wires:
  Product1/1 -> Pw_CellLoss/1  "Pw_LossCell"
  DOD->SOC/1 -> Resistance/1, Stop Function/2(Rt_SOC)
  Resistance/1 -> Product2/1
  I_cell [A]/1 -> State of charge calculation/1(I_cell [A]), Product1/2, Product2/2, Stop Function/1(I_cell [A])
  Product2/1 -> Add3/2, Product1/1  "U_DropCell"
  Rt_initSOC [-]/1 -> State of charge calculation/2(Rt_initSOC [-])
  Add3/1 -> U_cell [V]/1, Stop Function/3(U_Cell)
  Open-circuit voltage/1 -> Add3/1
  State of charge calculation/2(Rt_DOD [-]) -> Open-circuit voltage/1, DOD->SOC/1
  State of charge calculation/1(Rt_SOC [-]) -> Rt_SOC [-]/1

== system qss_tb_library/Energy Buffer/BEV Battery/Cell electrical model ==
  I_cell [A] : Inport
  Rt_initSOC [-] : Inport  Port=2
  Add3 : Sum
  DOD->SOC : Fcn  Expr=1-u(1)
  Open-circuit voltage : Lookup  InputValues=[-0.08,-0.03,0,0.005,0.025,0.05,0.085,0.155,0.25,0.3,0.34,0.365,0.395,0.41,0.5,0.52,0.62,0.7,0.73,0.76,0.8,0.82,0.83,0.85,0.89,0.9,0.91,0.92,0.935,0.95,0.965,0.98,0.99,0.995,1,1.011,1.015]  Table=[4.32,4.22,4.15,4.12,4.115,4.1,4.07,4.03,3.96,3.92,3.915,3.8937,3.8622,3.8537,3.7828,3.7672,3.7022,3.6562,3.6398,3.6098,3.4,3.3,3.2,3.18,3.17,3.15,3.1,3.1,3,2.95,2.8437,2.8437,2.8437,2.8437,2.8437,2.5,2]  LookUpMeth=Interpolation-Use End Values
  Product1 : Product  Inputs=**  RndMeth=Zero
  Product2 : Product  Inputs=**  RndMeth=Zero
  Resistance : Lookup  InputValues=[0,0.166,0.333,0.5,0.666,0.833,1]  Table=[0.01,0.005,0.002,0.0018,0.0015,0.0013,0.0011]
  State of charge calculation : Subsystem
  Stop Function : Subsystem
  Rt_SOC [-] : Outport
  U_cell [V] : Outport  Port=2
  Pw_CellLoss : Outport  Port=3
  wires:
  Product1/1 -> Pw_CellLoss/1  "Pw_LossCell"
  DOD->SOC/1 -> Resistance/1, Stop Function/2(Rt_SOC)
  Resistance/1 -> Product2/1
  I_cell [A]/1 -> State of charge calculation/1(I_cell [A]), Product1/2, Product2/2, Stop Function/1(I_cell [A])
  Product2/1 -> Add3/2, Product1/1  "U_DropCell"
  Rt_initSOC [-]/1 -> State of charge calculation/2(Rt_initSOC [-])
  Add3/1 -> U_cell [V]/1, Stop Function/3(U_Cell)
  Open-circuit voltage/1 -> Add3/1
  State of charge calculation/2(Rt_DOD [-]) -> Open-circuit voltage/1, DOD->SOC/1
  State of charge calculation/1(Rt_SOC [-]) -> Rt_SOC [-]/1

== system qss_tb_library/Energy Buffer/Battery Assignment/Cell electrical model ==
  I_cell [A] : Inport
  Rt_initSOC [-] : Inport  Port=2
  Add3 : Sum
  DOD->SOC : Fcn  Expr=1-u(1)
  Open-circuit voltage : Lookup  InputValues=[-0.08,-0.03,0,0.005,0.025,0.05,0.085,0.155,0.25,0.3,0.34,0.365,0.395,0.41,0.5,0.52,0.62,0.7,0.73,0.76,0.8,0.82,0.83,0.85,0.89,0.9,0.91,0.92,0.935,0.95,0.965,0.98,0.99,0.995,1,1.011,1.015]  Table=[4.32,4.22,4.15,4.12,4.115,4.1,4.07,4.03,3.96,3.92,3.915,3.8937,3.8622,3.8537,3.7828,3.7672,3.7022,3.6562,3.6398,3.6098,3.4,3.3,3.2,3.18,3.17,3.15,3.1,3.1,3,2.95,2.8437,2.8437,2.8437,2.8437,2.8437,2.5,2]  LookUpMeth=Interpolation-Use End Values
  Product1 : Product  Inputs=**  RndMeth=Zero
  Product2 : Product  Inputs=**  RndMeth=Zero
  Resistance : Lookup  InputValues=[0,0.16666666666666666,0.3333333333333333,0.5,0.6666666666666666,0.8333333333333334,1]  Table=[0.024012,0.0100,0.0075,0.00375,0.0022500000000000003,0.0015,0.0011250000000000001]
  State of charge calculation : Subsystem
  Stop Function : Subsystem
  Rt_SOC [-] : Outport
  U_cell [V] : Outport  Port=2
  Pw_CellLoss : Outport  Port=3
  wires:
  Product1/1 -> Pw_CellLoss/1  "Pw_LossCell"
  DOD->SOC/1 -> Resistance/1, Stop Function/2(Rt_SOC)
  Resistance/1 -> Product2/1
  I_cell [A]/1 -> State of charge calculation/1(I_cell [A]), Product1/2, Product2/2, Stop Function/1(I_cell [A])
  Product2/1 -> Add3/2, Product1/1  "U_DropCell"
  Rt_initSOC [-]/1 -> State of charge calculation/2(Rt_initSOC [-])
  Add3/1 -> U_cell [V]/1, Stop Function/3(U_Cell)
  Open-circuit voltage/1 -> Add3/1
  State of charge calculation/2(Rt_DOD [-]) -> Open-circuit voltage/1, DOD->SOC/1
  State of charge calculation/1(Rt_SOC [-]) -> Rt_SOC [-]/1

== system qss_tb_library/Energy Buffer/HEV Battery/Cell electrical model ==
  I_cell [A] : Inport
  Rt_initSOC [-] : Inport  Port=2
  Add3 : Sum
  DOD->SOC : Fcn  Expr=1-u(1)
  Open-circuit voltage : Lookup  InputValues=[-0.08,-0.03,0,0.005,0.025,0.05,0.085,0.155,0.25,0.3,0.34,0.365,0.395,0.41,0.5,0.52,0.62,0.7,0.73,0.76,0.8,0.82,0.83,0.85,0.89,0.9,0.91,0.92,0.935,0.95,0.965,0.98,0.99,0.995,1,1.011,1.015]  Table=[4.32,4.22,4.15,4.12,4.115,4.1,4.07,4.03,3.96,3.92,3.915,3.8937,3.8622,3.8537,3.7828,3.7672,3.7022,3.6562,3.6398,3.6098,3.4,3.3,3.2,3.18,3.17,3.15,3.1,3.1,3,2.95,2.8437,2.8437,2.8437,2.8437,2.8437,2.5,2]  LookUpMeth=Interpolation-Use End Values
  Product1 : Product  Inputs=**  RndMeth=Zero
  Product2 : Product  Inputs=**  RndMeth=Zero
  Resistance : Lookup  InputValues=[0,0.16666666666666666,0.3333333333333333,0.5,0.6666666666666666,0.8333333333333334,1]  Table=0.75*[0.024012,0.0100,0.0075,0.00375,0.0022500000000000003,0.0015,0.0011250000000000001]
  State of charge calculation : Subsystem
  Stop Function : Subsystem
  Rt_SOC [-] : Outport
  U_cell [V] : Outport  Port=2
  Pw_CellLoss : Outport  Port=3
  wires:
  Product1/1 -> Pw_CellLoss/1  "Pw_LossCell"
  DOD->SOC/1 -> Resistance/1, Stop Function/2(Rt_SOC)
  Resistance/1 -> Product2/1
  I_cell [A]/1 -> State of charge calculation/1(I_cell [A]), Product1/2, Product2/2, Stop Function/1(I_cell [A])
  Product2/1 -> Add3/2, Product1/1  "U_DropCell"
  Rt_initSOC [-]/1 -> State of charge calculation/2(Rt_initSOC [-])
  Add3/1 -> U_cell [V]/1, Stop Function/3(U_Cell)
  Open-circuit voltage/1 -> Add3/1
  State of charge calculation/2(Rt_DOD [-]) -> Open-circuit voltage/1, DOD->SOC/1
  State of charge calculation/1(Rt_SOC [-]) -> Rt_SOC [-]/1

== system qss_tb_library/Energy Buffer/PHEV Battery/Cell electrical model ==
  I_cell [A] : Inport
  Rt_initSOC [-] : Inport  Port=2
  Add3 : Sum
  DOD->SOC : Fcn  Expr=1-u(1)
  Open-circuit voltage : Lookup  InputValues=[-0.08,-0.03,0,0.005,0.025,0.05,0.085,0.155,0.25,0.3,0.34,0.365,0.395,0.41,0.5,0.52,0.62,0.7,0.73,0.76,0.8,0.82,0.83,0.85,0.89,0.9,0.91,0.92,0.935,0.95,0.965,0.98,0.99,0.995,1,1.011,1.015]  Table=[4.32,4.22,4.15,4.12,4.115,4.1,4.07,4.03,3.96,3.92,3.915,3.8937,3.8622,3.8537,3.7828,3.7672,3.7022,3.6562,3.6398,3.6098,3.4,3.3,3.2,3.18,3.17,3.15,3.1,3.1,3,2.95,2.8437,2.8437,2.8437,2.8437,2.8437,2.5,2]  LookUpMeth=Interpolation-Use End Values
  Product1 : Product  Inputs=**  RndMeth=Zero
  Product2 : Product  Inputs=**  RndMeth=Zero
  Resistance : Lookup  InputValues=[0,0.16666666666666666,0.3333333333333333,0.5,0.6666666666666666,0.8333333333333334,1]  Table=0.5*[0.024012,0.0100,0.0075,0.00375,0.0022500000000000003,0.0015,0.0011250000000000001]
  State of charge calculation : Subsystem
  Stop Function : Subsystem
  Rt_SOC [-] : Outport
  U_cell [V] : Outport  Port=2
  Pw_CellLoss : Outport  Port=3
  wires:
  Product1/1 -> Pw_CellLoss/1  "Pw_LossCell"
  DOD->SOC/1 -> Resistance/1, Stop Function/2(Rt_SOC)
  Resistance/1 -> Product2/1
  I_cell [A]/1 -> State of charge calculation/1(I_cell [A]), Product1/2, Product2/2, Stop Function/1(I_cell [A])
  Product2/1 -> Add3/2, Product1/1  "U_DropCell"
  Rt_initSOC [-]/1 -> State of charge calculation/2(Rt_initSOC [-])
  Add3/1 -> U_cell [V]/1, Stop Function/3(U_Cell)
  Open-circuit voltage/1 -> Add3/1
  State of charge calculation/2(Rt_DOD [-]) -> Open-circuit voltage/1, DOD->SOC/1
  State of charge calculation/1(Rt_SOC [-]) -> Rt_SOC [-]/1
